simulink model "AIN_1x_C"  (R2018b)
settings: Solver=ode23t  StartTime=0.0  StopTime=0.5  RelTol=1e-3
undefined symbols (not defined in the file): DiscIntNeverNeededParam
libraries: powerlib x15, powerlib_meascontrol x2
settings Model: Creator=K2  LastModifiedBy=VID Company

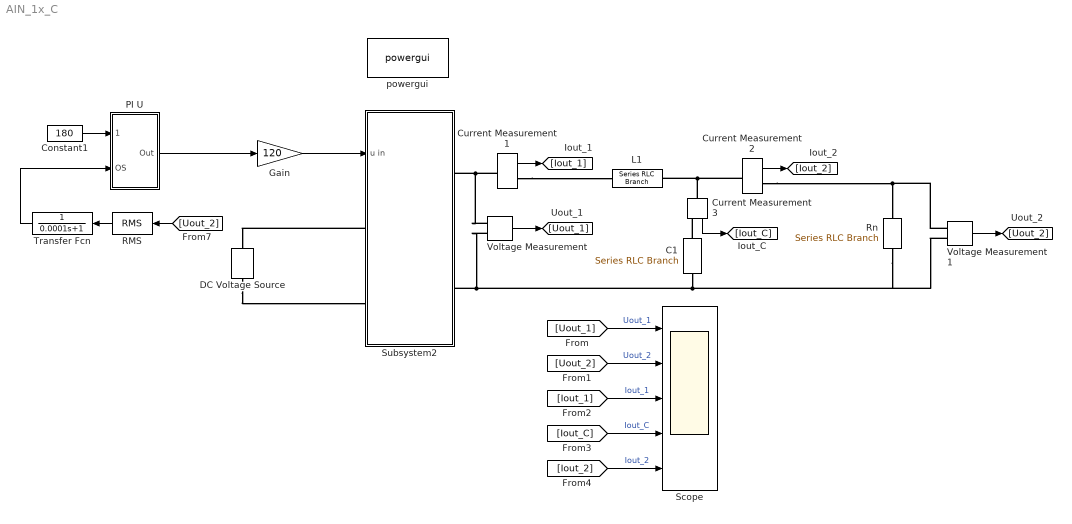
== system AIN_1x_C ==
  C1 : powerlib/Elements/Series RLC Branch  LConnTagsString=__new0  RConnTagsString=__new0  BranchType=RC  Resistance=0.050  Inductance=1e-3  SetiL0=off  InitialCurrent=0  Capacitance=50e-6  Setx0=off  InitialVoltage=0  Measurements=None
  Constant1 : Constant  Value=180  SampleTime=1e-6
  Current Measurement1 : powerlib/Measurements/Current Measurement  PhasorSimulation=off  OutputType=Complex  PSBequivalent=0
  Current Measurement2 : powerlib/Measurements/Current Measurement  PhasorSimulation=off  OutputType=Complex  PSBequivalent=0
  Current Measurement3 : powerlib/Measurements/Current Measurement  PhasorSimulation=off  OutputType=Complex  PSBequivalent=0
  DC Voltage Source : powerlib/Electrical Sources/DC Voltage Source  Amplitude=550  Measurements=None
  Gain : Gain  Gain=120
  L1 : powerlib/Elements/Series RLC Branch  LConnTagsString=__new0  RConnTagsString=__new0  BranchType=RL  Resistance=0.1  Inductance=0.3e-3  SetiL0=off  InitialCurrent=0  Capacitance=10e-3  Setx0=off  InitialVoltage=0  Measurements=None
  PI U : Subsystem
  RMS : powerlib_meascontrol/Measurements/RMS  TrueRMS=off  Freq=50  RMSInit=0  Ts=0
  Rn : powerlib/Elements/Series RLC Branch  LConnTagsString=__new0  RConnTagsString=__new0  BranchType=RL  Resistance=2  Inductance=0.001e-3  SetiL0=off  InitialCurrent=0  Capacitance=50e-6  Setx0=off  InitialVoltage=0  Measurements=None
  Scope : Scope  NumInputPorts=5
  Subsystem2 : Subsystem
  Transfer Fcn : TransferFcn  Denominator=[0.0001 1]
  Voltage Measurement : powerlib/Measurements/Voltage Measurement  PhasorSimulation=off  OutputType=Complex  PSBequivalent=0
  Voltage Measurement1 : powerlib/Measurements/Voltage Measurement  PhasorSimulation=off  OutputType=Complex  PSBequivalent=0
  powergui : powerlib/powergui  Priority=1  SimulationMode=Discrete  SampleTime=1e-6  frequency=60  Iterations=50  frequencyindice=0  Pbase=100e6  ErrMax=1e-4  UnitsV=kV  UnitsW=MW  buscounter=0  FunctionMessages=off  echomessages=off  EnableUseOfTLC=off  CurrentSourceSwitches=off  DisableSnubberDevices=off  DisableRonSwitches=off  DisableVfSwitches=off  DisplayEquations=off  SolverType=Tustin/Backward Euler (TBE)  Interpol=off  ExternalGateDelay=off  methode=off  Ts=100  x0status=blocks  SPID=on  SwTol=0  HookPort=off  RestoreLinks=warning  ResistiveCurrentMeasurement=off  Frange=[0:2:500]  Ylog=off  Xlog=on  ShowGrid=off  save=off  variable=ZData  structure=logsout  ZoomFFT=off  StartTime=0.4  cycles=4  DisplayStyle=1  fundamental=50  FreqAxis=off  MaxFrequency=20000  frequencyindicesteady=1  RmsSteady=1  display=off
  wires:
  Voltage Measurement/1 -> [Uout_1]
  Current Measurement1/1 -> [Iout_1]
  Current Measurement2/1 -> [Iout_2]
  Voltage Measurement1/1 -> [Uout_2]
  Current Measurement3/1 -> [Iout_C]
  [Uout_1] -> Scope/1  "Uout_1"
  [Iout_1] -> Scope/3  "Iout_1"
  [Uout_2] -> Scope/2  "Uout_2"
  [Iout_C] -> Scope/4  "Iout_C"
  [Iout_2] -> Scope/5  "Iout_2"
  Constant1/1 -> PI U/1(Zad)
  [Uout_2] -> RMS/1
  RMS/1 -> Transfer Fcn/1
  Gain/1 -> Subsystem2/1(u in)
  PI U/1(Out) -> Gain/1
  Transfer Fcn/1 -> PI U/2(OS)
  connections:
  DC Voltage Source/LConn1 -- Subsystem2/LConn2
  Voltage Measurement/LConn1 -- Current Measurement1/LConn1 -- Subsystem2/RConn1
  Current Measurement2/LConn1 -- L1/RConn1 -- Current Measurement3/LConn1
  C1/RConn1 -- Rn/RConn1 -- Voltage Measurement1/LConn2 -- Voltage Measurement/LConn2 -- Subsystem2/RConn2
  Subsystem2/LConn1 -- DC Voltage Source/RConn1
  Current Measurement1/RConn1 -- L1/LConn1
  Current Measurement2/RConn1 -- Rn/LConn1 -- Voltage Measurement1/LConn1
  C1/LConn1 -- Current Measurement3/RConn1

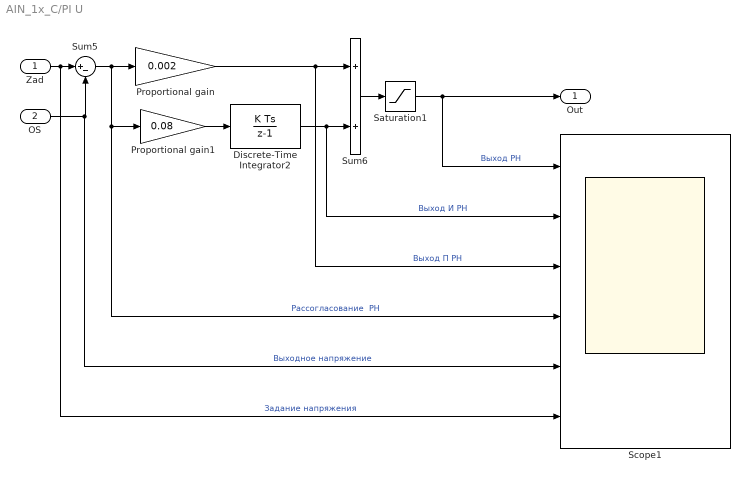
== system AIN_1x_C/PI U ==
  Zad : Inport
  OS : Inport  Port=2
  Discrete-Time Integrator2 : DiscreteIntegrator  SampleTime=-1  LimitOutput=on  UpperSaturationLimit=1  LowerSaturationLimit=0  ICPrevOutput=DiscIntNeverNeededParam  ICPrevScaledInput=DiscIntNeverNeededParam
  Proportional gain : Gain  Gain=0.002  SaturateOnIntegerOverflow=on  OutDataTypeStr=Inherit: Same as input  ParamDataTypeStr=Inherit: Same as input
  Proportional gain1 : Gain  Gain=0.08  SaturateOnIntegerOverflow=on  OutDataTypeStr=Inherit: Same as input  ParamDataTypeStr=Inherit: Same as input
  Saturation1 : Saturate  UpperLimit=1  LowerLimit=0
  Scope1 : Scope  NumInputPorts=6
  Sum5 : Sum  Inputs=|+-  SaturateOnIntegerOverflow=on  InputSameDT=on  OutDataTypeStr=Inherit: Same as first input
  Sum6 : Sum  SaturateOnIntegerOverflow=on  InputSameDT=on  OutDataTypeStr=Inherit: Same as first input
  Out : Outport
  wires:
  Proportional gain/1 -> Scope1/3, Sum6/1  "Выход П РН"
  Discrete-Time Integrator2/1 -> Sum6/2, Scope1/2  "Выход И РН"
  OS/1 -> Scope1/5, Sum5/2  "Выходное напряжение"
  Zad/1 -> Scope1/6, Sum5/1  "Задание напряжения"
  Sum5/1 -> Proportional gain1/1, Scope1/4, Proportional gain/1  "Рассогласование  РН"
  Sum6/1 -> Saturation1/1
  Saturation1/1 -> Out/1, Scope1/1  "Выход РН"
  Proportional gain1/1 -> Discrete-Time Integrator2/1

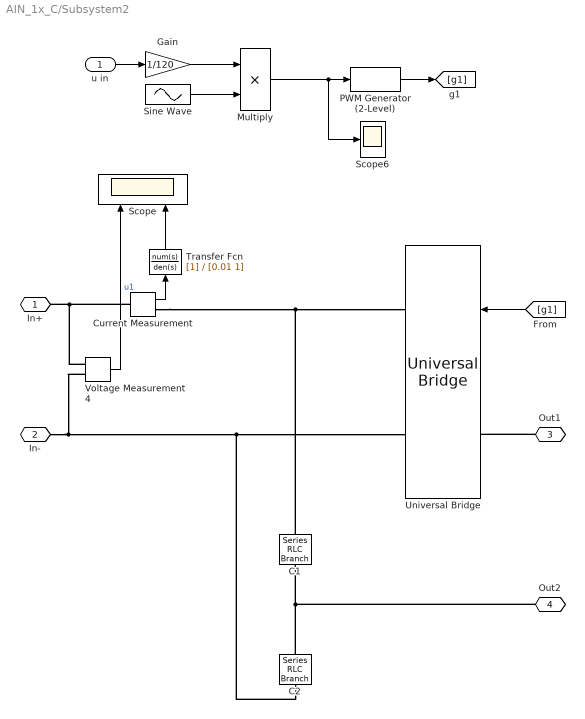
== system AIN_1x_C/Subsystem2 ==
  u in : Inport
  C1 : powerlib/Elements/Series RLC Branch  LConnTagsString=__new0  RConnTagsString=__new0  BranchType=RC  Resistance=0.020  Inductance=1e-3  SetiL0=off  InitialCurrent=0  Capacitance=10e-3  Setx0=off  InitialVoltage=0  Measurements=None
  C2 : powerlib/Elements/Series RLC Branch  LConnTagsString=__new0  RConnTagsString=__new0  BranchType=RC  Resistance=0.020  Inductance=1e-3  SetiL0=off  InitialCurrent=0  Capacitance=10e-3  Setx0=off  InitialVoltage=0  Measurements=None
  Current Measurement : powerlib/Measurements/Current Measurement  PhasorSimulation=off  OutputType=Complex  PSBequivalent=0
  Gain : Gain  Gain=1/120
  Multiply : Product
  PWM Generator (2-Level) : powerlib_meascontrol/Pulse & Signal Generators/PWM Generator (2-Level)  ModulatorType=Single-phase half-bridge (2 pulses)  ModulatorMode=Unsynchronized  Fc=8000  Pc=0  nF=27  MinMax="[ -1  1 ]"  SamplingTechnique=Natural  ModulatingSignals=off  m=0.8  Freq=60  Phase=0  Ts=0  ShowCarrierOutport=off
      settings: SourceProductName=Simscape Power Systems
  Scope : Scope  NumInputPorts=2
  Scope6 : Scope
  Sine Wave : Sin  Amplitude=0.95  Frequency=50*2*pi  SampleTime=0
  Transfer Fcn : TransferFcn  Denominator=[0.01 1]
  Universal Bridge : powerlib/Power Electronics/Universal Bridge  Arms=1  SnubberResistance=1e5  SnubberCapacitance=inf  Device=IGBT / Diodes  Ron=5e-3  Lon=0  ForwardVoltages="[  1.5  1  ]"  ForwardVoltage=0  GTOparameters=[ 10e-6 , 20e-6 ]  IGBTparameters=[ 1e-6 , 2e-6 ]  Measurements=Device currents  Measurements_2=None  converterType=Rectifier
  Voltage Measurement4 : powerlib/Measurements/Voltage Measurement  PhasorSimulation=off  OutputType=Complex  PSBequivalent=0
  In+ : PMIOPort  Side=Left
  In- : PMIOPort  Port=2  Side=Left
  Out1 : PMIOPort  Port=3  Side=Right
  Out2 : PMIOPort  Port=4  Side=Right
  wires:
  [g1] -> Universal Bridge/1
  PWM Generator (2-Level)/1 -> [g1]
  Gain/1 -> Multiply/1
  u in/1 -> Gain/1
  Multiply/1 -> Scope6/1, PWM Generator (2-Level)/1
  Sine Wave/1 -> Multiply/2
  Current Measurement/1 -> Transfer Fcn/1
  Voltage Measurement4/1 -> Scope/1  "u1"
  Transfer Fcn/1 -> Scope/2
  connections:
  Current Measurement/LConn1 -- Voltage Measurement4/LConn1 -- In+/RConn1
  Out1/RConn1 -- Universal Bridge/LConn1
  In-/RConn1 -- Voltage Measurement4/LConn2 -- C2/RConn1 -- Universal Bridge/RConn2
  Current Measurement/RConn1 -- C1/LConn1 -- Universal Bridge/RConn1
  C2/LConn1 -- Out2/RConn1 -- C1/RConn1
